simulink model "L7_sim2"  (R2024b)
settings: Solver=VariableStepAuto  StartTime=0.0  StopTime=100  RelTol=1e-3
values from neighbouring files (symbols this model uses):
  a = ((Ra+Rp)/2)*1e3    (= 9128137)    [Task1.m]    (also in Task2.m; Task3.m = 6878137)
  A_0 = eye(3)    [Task1.m]    (also in Task2.m; Task3.m = R_z_0 * R_x_0)
  e = (Ra-Rp)/(Ra+Rp)    (= 0.246490603723)    [Task1.m]    (also in Task2.m; Task3.m = 0)
  eps_rad = deg2rad(23.45)    [Task1.m]    (also in Task2.m; Task3.m)
  I = diag([Ix(5), Iy(5), Iz(5)])    [Task1.m]    (also in Task2.m = J_depl; Task3.m = J_depl)
  i = deg2rad(28.5)    [Task1.m]    (also in Task2.m; Task3.m)
  n = sqrt(G*M_t/(a/1e3)^3)    [Task1.m]    (also in Task2.m; Task3.m)
  n_sun = 2*pi/T_year    (= 1.99102127766e-07)    [Task1.m]    (also in Task2.m; Task3.m)
  orthonormalize = 0    [Task1.m]    (also in Task2.m; Task3.m)
  r_cm = [0; 0; 0.02]    [Task2.m]    (also in Task3.m)
  w_0 = [1e-6, 1e-6, n]'    [Task1.m]    (also in Task2.m; Task3.m = [1e-6, 1e-6, theta_dot_0]')
libraries: matrix_library x1
settings Model: Creator=alejandromunozvazquez  LastModifiedBy=alejandromunozvazquez

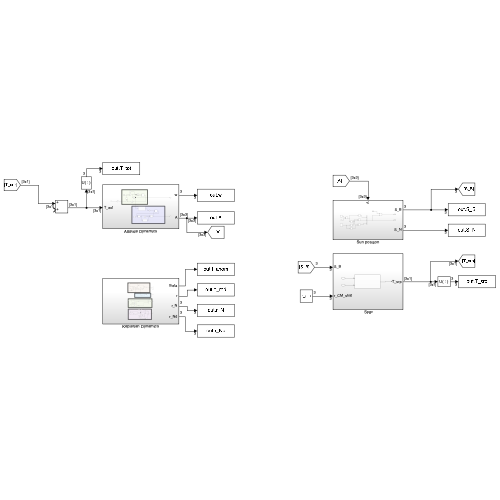
[thumbnail: Simulink's stored preview of the top-level diagram]
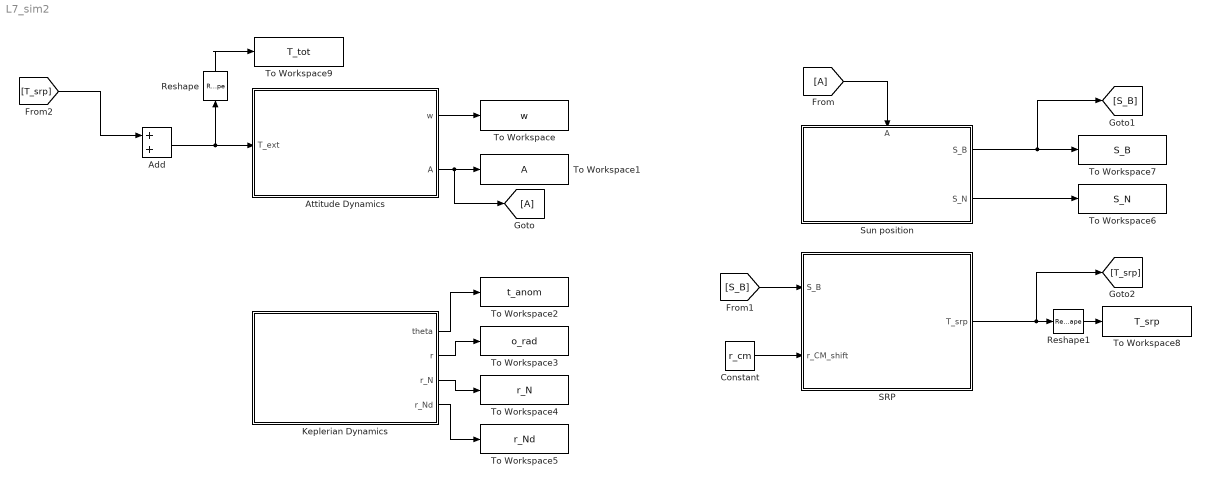
== system L7_sim2 ==
  " SRP" : Subsystem
  Add : Sum
  Attitude Dynamics : Subsystem
  Constant : Constant  Value=r_cm
  From : From
  Goto : Goto
  Keplerian Dynamics : Subsystem
  Reshape : Reshape
  Reshape1 : Reshape
  Sun position : Subsystem
      settings: PortSchema="{\"entries\":[{\"content\":{\"sides\":[{\"content\":{},\"type\":\"ConnectorPlacement.EquallySpacedRectSide\",\"uuid\":\"21a6b8b0-bde3-49fd-9e9b-cf3d5081f5fb\"},{\"content\":{\"connectorIds\":[\"Out1\",\"Out2\"],\"side\":\"RIGHT\"},\"type\":\"ConnectorPlacement.EquallySpacedRectSide\",\"uuid\":\"f4269799-f186-41ab-bed9-285a1d71e8b2\"},{\"content\":{\"connectorIds\":[\"In1\"],\"side\":\"TOP\"},\"type\":\"ConnectorPlacement.EquallySpacedRectSide\",\"uuid\":\"cf7f5999-454e-479f-928a-3f86d9304e37\"}]},\"type\":\"ConnectorPlacement.EquallySpacedConnector\",\"uuid\":\"7fd823eb-300a-45c2-b517-5238835a94d5\"}],\"packageUris\":[\"http://schema.mathworks.com/mf0/Connector/R2020b\"],\"version\":\"1.0\"}"
  To Workspace : ToWorkspace  VariableName=w  SampleTime=-1
  To Workspace1 : ToWorkspace  VariableName=A  SampleTime=-1
  To Workspace2 : ToWorkspace  VariableName=t_anom  SampleTime=-1
  To Workspace3 : ToWorkspace  VariableName=o_rad  SampleTime=-1
  To Workspace4 : ToWorkspace  VariableName=r_N  SampleTime=-1
  To Workspace5 : ToWorkspace  VariableName=r_Nd  SampleTime=-1
  To Workspace6 : ToWorkspace  VariableName=S_N  SampleTime=-1
  To Workspace7 : ToWorkspace  VariableName=S_B  SampleTime=-1
  To Workspace8 : ToWorkspace  VariableName=T_srp  SampleTime=-1
  To Workspace9 : ToWorkspace  VariableName=T_tot  SampleTime=-1
  wires:
  Attitude Dynamics/1(w) -> To Workspace/1
  Attitude Dynamics/2(A) -> Goto/1, To Workspace1/1
  Keplerian Dynamics/1(theta) -> To Workspace2/1
  Keplerian Dynamics/2(r) -> To Workspace3/1
  Keplerian Dynamics/3(r_N) -> To Workspace4/1
  Keplerian Dynamics/4(r_Nd) -> To Workspace5/1
  Sun position/1(S_B) -> [S_B], To Workspace7/1
  Sun position/2(S_N) -> To Workspace6/1
  From/1 -> Sun position/1(A)
  [S_B] -> " SRP"/1(S_B)
  Constant/1 -> " SRP"/2(r_CM_shift)
  " SRP"/1(T_srp) -> [T_srp], Reshape1/1
  [T_srp] -> Add/1
  Add/1 -> Reshape/1, Attitude Dynamics/1(T_ext)
  Reshape/1 -> To Workspace9/1
  Reshape1/1 -> To Workspace8/1

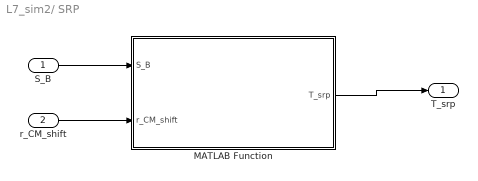
== system L7_sim2/ SRP ==
  S_B : Inport
  r_CM_shift : Inport  Port=2
  MATLAB Function : MATLAB Function  TreatAsAtomicUnit=on
  T_srp : Outport
  wires:
  S_B/1 -> MATLAB Function/1(S_B)
  r_CM_shift/1 -> MATLAB Function/2(r_CM_shift)
  MATLAB Function/1(T_srp) -> T_srp/1

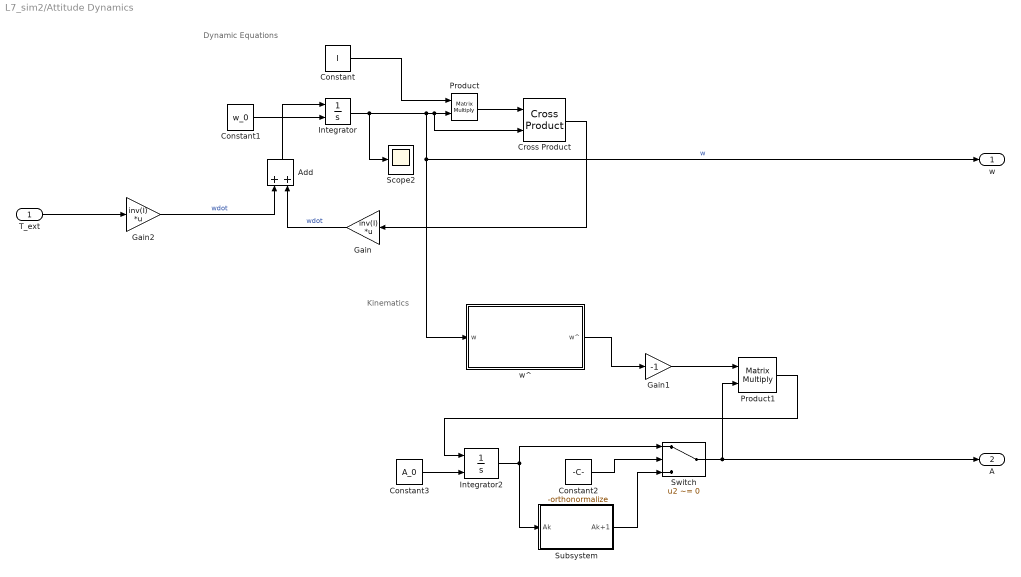
== system L7_sim2/Attitude Dynamics ==
  note: Kinematics
  note: Dynamic Equations
  T_ext : Inport
  Add : Sum
  Constant : Constant  Value=I
  Constant1 : Constant  Value=w_0
  Constant2 : Constant  Value=-orthonormalize
  Constant3 : Constant  Value=A_0
  Cross Product : matrix_library/Cross Product
  Gain : Gain  Gain=inv(I)  Multiplication=Matrix(K*u) (u vector)
  Gain1 : Gain  Gain=-1
  Gain2 : Gain  Gain=inv(I)  Multiplication=Matrix(K*u) (u vector)
  Integrator : Integrator  InitialConditionSource=external
  Integrator2 : Integrator  InitialConditionSource=external
  Product : Product  Multiplication=Matrix(*)
  Product1 : Product  Multiplication=Matrix(*)
  Scope2 : Scope
  Subsystem : Subsystem
  Switch : Switch  Criteria=u2 ~= 0  SaturateOnIntegerOverflow=off  InputSameDT=off
  "w^ " : Subsystem
  w : Outport
  A : Outport  Port=2
  wires:
  "w^ "/1(w^) -> Gain1/1
  Constant/1 -> Product/1
  Constant2/1 -> Switch/2
  Product/1 -> Cross Product/1
  Switch/1 -> A/1, Product1/2
  Gain/1 -> Add/2  "wdot"
  Product1/1 -> Integrator2/1
  Cross Product/1 -> Gain/1
  Constant3/1 -> Integrator2/2
  Integrator/1 -> Scope2/1, Product/2, Cross Product/2, w/1, "w^ "/1(w)  "w"
  Constant1/1 -> Integrator/2
  Gain1/1 -> Product1/1
  Subsystem/1(Ak+1) -> Switch/3
  Integrator2/1 -> Subsystem/1(Ak), Switch/1
  T_ext/1 -> Gain2/1
  Gain2/1 -> Add/1  "wdot"
  Add/1 -> Integrator/1

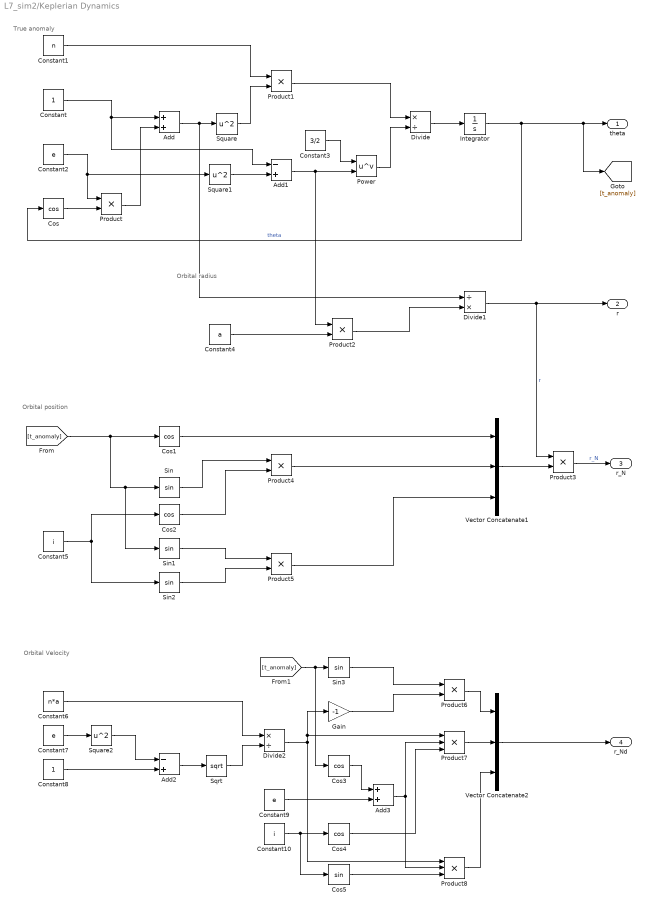
== system L7_sim2/Keplerian Dynamics ==
  note: Orbital Velocity
  note: True anomaly
  note: Orbital radius
  note: Orbital position
  Add : Sum
  Add1 : Sum  Inputs=-+
  Add2 : Sum  Inputs=-+
  Add3 : Sum
  Constant : Constant
  Constant1 : Constant  Value=n
  Constant10 : Constant  Value=i
  Constant2 : Constant  Value=e
  Constant3 : Constant  Value=3/2
  Constant4 : Constant  Value=a
  Constant5 : Constant  Value=i
  Constant6 : Constant  Value=n*a
  Constant7 : Constant  Value=e
  Constant8 : Constant
  Constant9 : Constant  Value=e
  Cos{,1..4} (5 alike) : Trigonometry  Operator=cos
  Cos5 : Trigonometry
  Divide : Product  Inputs=*/
  Divide1 : Product  Inputs=/*
  Divide2 : Product  Inputs=*/
  Gain : Gain  Gain=-1
  Integrator : Integrator
  Power : Math  Operator=pow
  Product{,1..6} (7 alike) : Product
  Product7 : Product  Inputs=3
  Product8 : Product  Inputs=3
  Sin{,1..3} (4 alike) : Trigonometry
  Sqrt : Sqrt
  Square : Math  Operator=square
  Square1 : Math  Operator=square
  Square2 : Math  Operator=square
  Vector Concatenate1 : Concatenate  NumInputs=3
  Vector Concatenate2 : Concatenate  NumInputs=3
  theta : Outport
  r : Outport  Port=2
  r_N : Outport  Port=3
  r_Nd : Outport  Port=4
  wires:
  Integrator/1 -> Cos/1, [t_anomaly], theta/1  "theta"
  Constant2/1 -> Product/1, Square1/1
  Cos/1 -> Product/2
  Product/1 -> Add/2
  Constant/1 -> Add1/1, Add/1
  Constant1/1 -> Product1/1
  Add/1 -> Divide1/1, Square/1
  Square/1 -> Product1/2
  Product1/1 -> Divide/1
  Square1/1 -> Add1/2
  Add1/1 -> Power/2, Product2/1
  Constant3/1 -> Power/1
  Power/1 -> Divide/2
  Divide/1 -> Integrator/1
  Constant4/1 -> Product2/2
  Product2/1 -> Divide1/2
  Divide1/1 -> r/1, Product3/1  "r"
  [t_anomaly] -> Sin1/1, Sin/1, Cos1/1
  Product3/1 -> r_N/1  "r_N"
  Vector Concatenate1/1 -> Product3/2
  Cos1/1 -> Vector Concatenate1/1
  Constant5/1 -> Sin2/1, Cos2/1
  Cos2/1 -> Product4/2
  Sin/1 -> Product4/1
  Product4/1 -> Vector Concatenate1/2
  Sin1/1 -> Product5/1
  Sin2/1 -> Product5/2
  Product5/1 -> Vector Concatenate1/3
  Constant7/1 -> Square2/1
  Square2/1 -> Add2/1
  Constant8/1 -> Add2/2
  Add2/1 -> Sqrt/1
  Sqrt/1 -> Divide2/2
  Constant6/1 -> Divide2/1
  Product6/1 -> Vector Concatenate2/1
  [t_anomaly] -> Cos3/1, Sin3/1
  Gain/1 -> Product6/2
  Divide2/1 -> Product8/1, Product7/1, Gain/1
  Sin3/1 -> Product6/1
  Cos3/1 -> Add3/1
  Constant9/1 -> Add3/2
  Constant10/1 -> Cos5/1, Cos4/1
  Add3/1 -> Product8/2, Product7/2
  Cos4/1 -> Product7/3
  Product7/1 -> Vector Concatenate2/2
  Cos5/1 -> Product8/3
  Product8/1 -> Vector Concatenate2/3
  Vector Concatenate2/1 -> r_Nd/1

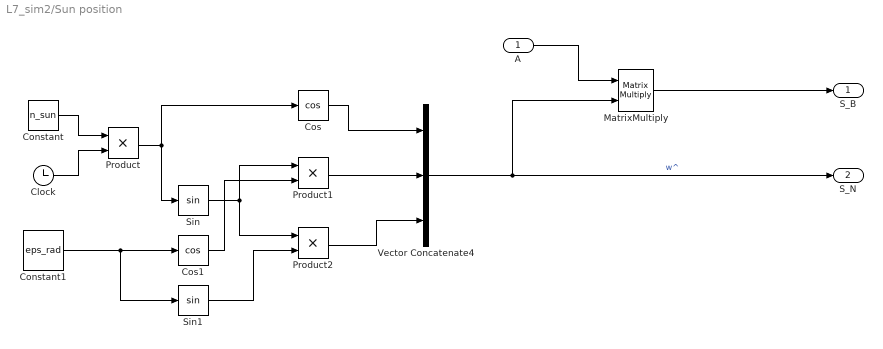
== system L7_sim2/Sun position ==
  A : Inport
  Clock : Clock
  Constant : Constant  Value=n_sun
  Constant1 : Constant  Value=eps_rad
  Cos : Trigonometry  Operator=cos
  Cos1 : Trigonometry  Operator=cos
  MatrixMultiply : Product  Multiplication=Matrix(*)
  Product : Product
  Product1 : Product
  Product2 : Product
  Sin : Trigonometry
  Sin1 : Trigonometry
  Vector Concatenate4 : Concatenate  NumInputs=3  ConcatenateDimension=2
  S_B : Outport
  S_N : Outport  Port=2
  wires:
  Product1/1 -> Vector Concatenate4/2
  MatrixMultiply/1 -> S_B/1
  Cos/1 -> Vector Concatenate4/1
  Product/1 -> Sin/1, Cos/1
  Product2/1 -> Vector Concatenate4/3
  Constant/1 -> Product/1
  Vector Concatenate4/1 -> S_N/1, MatrixMultiply/2  "w^"
  A/1 -> MatrixMultiply/1
  Clock/1 -> Product/2
  Sin/1 -> Product1/1, Product2/1
  Constant1/1 -> Sin1/1, Cos1/1
  Sin1/1 -> Product2/2
  Cos1/1 -> Product1/2

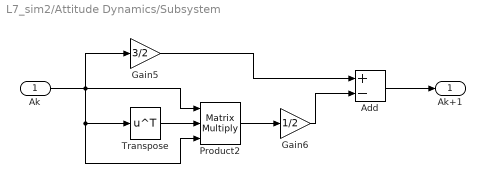
== system L7_sim2/Attitude Dynamics/Subsystem ==
  Ak : Inport
  Add : Sum  Inputs=+-
  Gain5 : Gain  Gain=3/2
  Gain6 : Gain  Gain=1/2
  Product2 : Product  Inputs=3  Multiplication=Matrix(*)
  Transpose : Math  Operator=transpose
  Ak+1 : Outport
  wires:
  Gain5/1 -> Add/1
  Add/1 -> Ak+1/1
  Product2/1 -> Gain6/1
  Gain6/1 -> Add/2
  Transpose/1 -> Product2/2
  Ak/1 -> Product2/3, Transpose/1, Gain5/1, Product2/1

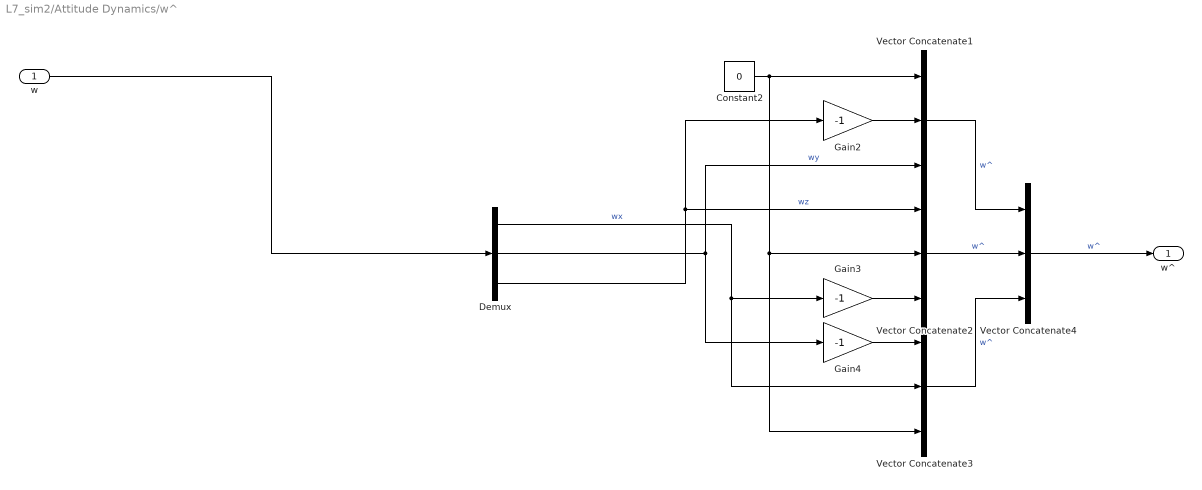
== system L7_sim2/Attitude Dynamics/w^  ==
  w : Inport
  Constant2 : Constant  Value=0
  Demux : Demux  Outputs=3
  Gain2 : Gain  Gain=-1
  Gain3 : Gain  Gain=-1
  Gain4 : Gain  Gain=-1
  Vector Concatenate1 : Concatenate  NumInputs=3  Mode=Multidimensional array
  Vector Concatenate2 : Concatenate  NumInputs=3  Mode=Multidimensional array
  Vector Concatenate3 : Concatenate  NumInputs=3  Mode=Multidimensional array
  Vector Concatenate4 : Concatenate  NumInputs=3  Mode=Multidimensional array  ConcatenateDimension=2
  w^ : Outport
  wires:
  w/1 -> Demux/1
  Vector Concatenate4/1 -> w^/1  "w^"
  Demux/2 -> Vector Concatenate1/3, Gain4/1  "wy"
  Vector Concatenate1/1 -> Vector Concatenate4/1  "w^"
  Demux/1 -> Vector Concatenate3/2, Gain3/1  "wx"
  Gain2/1 -> Vector Concatenate1/2
  Vector Concatenate3/1 -> Vector Concatenate4/3  "w^"
  Gain4/1 -> Vector Concatenate3/1
  Constant2/1 -> Vector Concatenate1/1, Vector Concatenate2/2, Vector Concatenate3/3
  Vector Concatenate2/1 -> Vector Concatenate4/2  "w^"
  Gain3/1 -> Vector Concatenate2/3
  Demux/3 -> Gain2/1, Vector Concatenate2/1  "wz"

== matlab function L7_sim2/ SRP/MATLAB Function ==
  data: S_B input; T_srp output; r_CM_shift input; satellite_data parameter
function T_srp = calculate_srp_torque(S_B, r_CM_shift, satellite_data)
    % S_B: Vector unitario al sol en Body Frame (3x1)
    % r_CM_shift: Desplazamiento del Centro de Masas (3x1) [m]
    % satellite_data: Estructura con los datos leídos del Excel
    
    % Constantes físicas
    Fe = 1358; % W/m^2
    c = 299792458; % m/s
    P = Fe / c; %
    
    T_srp = [0; 0; 0];
    num_faces = size(satellite_data.Normals, 2);

    for i = 1:num_faces
        N_Bi = satellite_data.Normals(:,i);
        r_Pi = satellite_data.Positions(:,i);
        Ai   = satellite_data.Areas(i);
        rs   = satellite_data.RhoS(i);
        rd   = satellite_data.RhoD(i);
        
        % Producto escalar para verificar iluminación
        cos_theta = dot(S_B, N_Bi);
        
        if cos_theta > 0
            % Cálculo de la fuerza Fi
            term1 = (1 - rs) * S_B;
            term2 = (2 * rs * cos_theta + (2/3) * rd) * N_Bi;
            Fi = -P * Ai * cos_theta * (term1 + term2);
            
            % Torque respecto al nuevo CM: (r_Pi - r_CM) x Fi
            T_srp = T_srp + cross(r_Pi - r_CM_shift, Fi);
        end
    end
end
